simulink model "GDPWM"  (R2023b)
settings: Solver=FixedStepAuto  StartTime=0.0  StopTime=0.08  FixedStep=1e-6  RelTol=1e-3
undefined symbols (not defined in the file): phase_angle
settings Model: Creator=user  LastModifiedBy=user

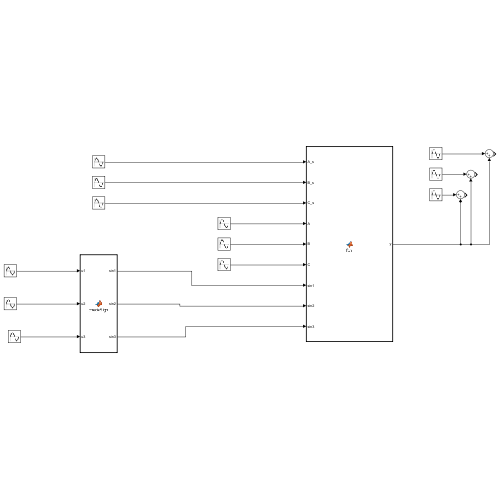
[thumbnail: Simulink's stored preview of the top-level diagram]
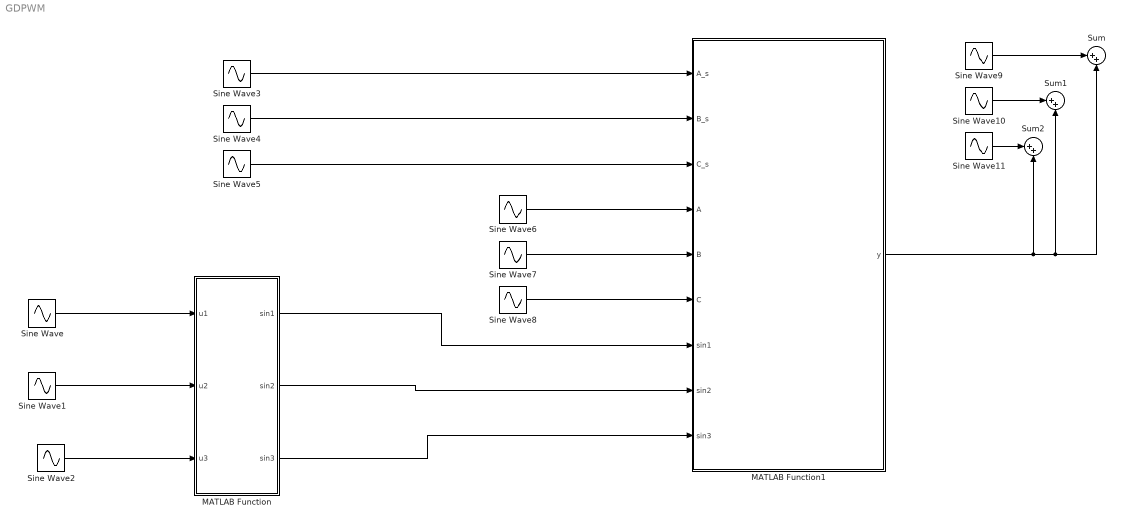
== system GDPWM ==
  MATLAB Function : MATLAB Function  TreatAsAtomicUnit=on
  MATLAB Function1 : MATLAB Function  TreatAsAtomicUnit=on
  Sine Wave : Sin  Frequency=2*pi*50  SampleTime=0
  Sine Wave1 : Sin  Frequency=2*pi*50  Phase=(2*pi/3)  SampleTime=0
  Sine Wave10 : Sin  Frequency=2*pi*50  Phase=(2*pi/3)  SampleTime=0
  Sine Wave11 : Sin  Frequency=2*pi*50  Phase=-2*pi/3  SampleTime=0
  Sine Wave2 : Sin  Frequency=2*pi*50  Phase=-2*pi/3  SampleTime=0
  Sine Wave3 : Sin  Frequency=2*pi*50  Phase=phase_angle  SampleTime=0
  Sine Wave4 : Sin  Frequency=2*pi*50  Phase=(2*pi/3)+phase_angle  SampleTime=0
  Sine Wave5 : Sin  Frequency=2*pi*50  Phase=-2*(pi/3)+phase_angle  SampleTime=0
  Sine Wave6 : Sin  Frequency=2*pi*50  SampleTime=0
  Sine Wave7 : Sin  Frequency=2*pi*50  Phase=(2*pi/3)  SampleTime=0
  Sine Wave8 : Sin  Frequency=2*pi*50  Phase=-2*pi/3  SampleTime=0
  Sine Wave9 : Sin  Frequency=2*pi*50  SampleTime=0
  Sum : Sum  Inputs=|++
  Sum1 : Sum  Inputs=|++
  Sum2 : Sum  Inputs=|++
  wires:
  Sine Wave/1 -> MATLAB Function/1(u1)
  Sine Wave1/1 -> MATLAB Function/2(u2)
  Sine Wave2/1 -> MATLAB Function/3(u3)
  Sine Wave3/1 -> MATLAB Function1/1(A_s)
  Sine Wave4/1 -> MATLAB Function1/2(B_s)
  Sine Wave5/1 -> MATLAB Function1/3(C_s)
  MATLAB Function/1(sin1) -> MATLAB Function1/7(sin1)
  Sine Wave6/1 -> MATLAB Function1/4(A)
  Sine Wave7/1 -> MATLAB Function1/5(B)
  Sine Wave8/1 -> MATLAB Function1/6(C)
  MATLAB Function/2(sin2) -> MATLAB Function1/8(sin2)
  MATLAB Function/3(sin3) -> MATLAB Function1/9(sin3)
  MATLAB Function1/1(y) -> Sum2/2, Sum1/2, Sum/2
  Sine Wave9/1 -> Sum/1
  Sine Wave10/1 -> Sum1/1
  Sine Wave11/1 -> Sum2/1

== matlab function GDPWM/MATLAB Function1 ==
  data: A_s input; B_s input; C_s input; A input; B input; C input; sin1 input; y output; sin2 input; sin3 input
function y = fcn(A_s, B_s, C_s, A, B, C, sin1, sin2, sin3)
z=0;
if(A_s>=B_s &&A_s>=C_s)
    z=sin1-A;
elseif(B_s>=A_s &&B_s>=C_s)
        z=sin2-B;
elseif(C_s>=A_s &&C_s>=B_s)
            z=sin3-C;
else
    z=min([A, B, C]);
end
            y = z;

== matlab function GDPWM/MATLAB Function ==
  data: sin1 output; u1 input; u2 input; sin2 output; u3 input; sin3 output
function [sin1, sin2, sin3] = checkSign(u1, u2, u3)
    sin1 = sign(u1);
    sin2 = sign(u2);
    sin3 = sign(u3);
end
